simulink model "Astrolab_jumeaunumerique_2015a_v21"  (R2015b)
settings: Solver=ode3  SolverMode=SingleTasking  StartTime=0.0  StopTime=10  RelTol=1e-3
model workspace (MAT data in the model file):
  Freq = Simulink.Parameter
  Freq.DataType = 'auto'
  Freq.Units = 'auto'
  Freq.DocUnits = 'Hz'
libraries: powerlib_meascontrol x2
settings Model: Creator=utilisateur  LastModifiedBy=utilisateur
settings DataIOCC: LimitDataPoints=off  ReturnWorkspaceOutputs=on
settings DebuggingCC: SFUnexpectedBacktrackingDiag=error  SFNoUnconditionalDefaultTransitionDiag=error
settings HardwareCC: ProdWordSize=32  ProdHWDeviceType=Specified
settings ModelReferenceCC: PropagateSignalLabelsOutOfModel=on
settings SFSimCC: SimUseLocalCustomCode=on
settings RTWCC: RTWUseLocalCustomCode=on
settings GRTTargetCC: TargetLangStandard=C99 (ISO)
settings ConfigComp: CovMetricSettings=dwe  CovHtmlReporting=off  CovSaveCumulativeToWorkspaceVar=off  CovSaveSingleToWorkspaceVar=off  CovModelRefEnable=Off  CovExternalEMLEnable=on
settings ConfigurationSet: Description=Simscape Multibody

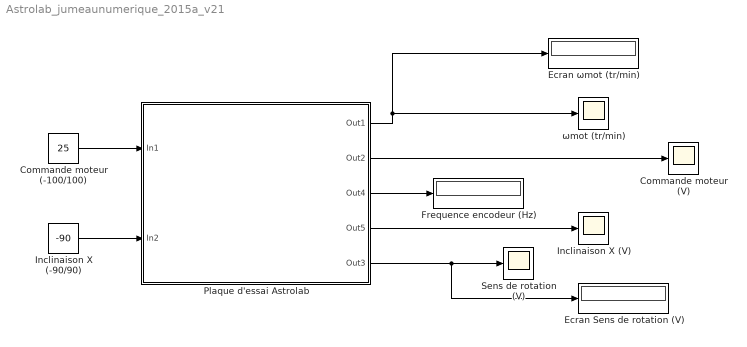
== system Astrolab_jumeaunumerique_2015a_v21 ==
  Commande moteur (-100/100) : Constant  Value=25
  Commande moteur (V) : Scope
  Ecran Sens de rotation (V) : Display
  Ecran ωmot (tr/min) : Display
  Frequence encodeur (Hz) : Display
  Inclinaison X (-90/90) : Constant  Value=-90
  Inclinaison X (V) : Scope
  Plaque d'essai Astrolab : Subsystem
      mask Display: image('plaque_astrolab.PNG')
  Sens de rotation (V) : Scope
  ωmot (tr/min) : Scope
  wires:
  Plaque d'essai Astrolab/1(Out1) -> Ecran ωmot (tr/min)/1, ωmot (tr/min)/1
  Plaque d'essai Astrolab/2(Out2) -> Commande moteur (V)/1
  Plaque d'essai Astrolab/3(Out4) -> Frequence encodeur (Hz)/1
  Plaque d'essai Astrolab/4(Out5) -> Inclinaison X (V)/1
  Inclinaison X (-90/90)/1 -> Plaque d'essai Astrolab/2(In2)
  Commande moteur (-100/100)/1 -> Plaque d'essai Astrolab/1(In1)
  Plaque d'essai Astrolab/5(Out3) -> Ecran Sens de rotation (V)/1, Sens de rotation (V)/1

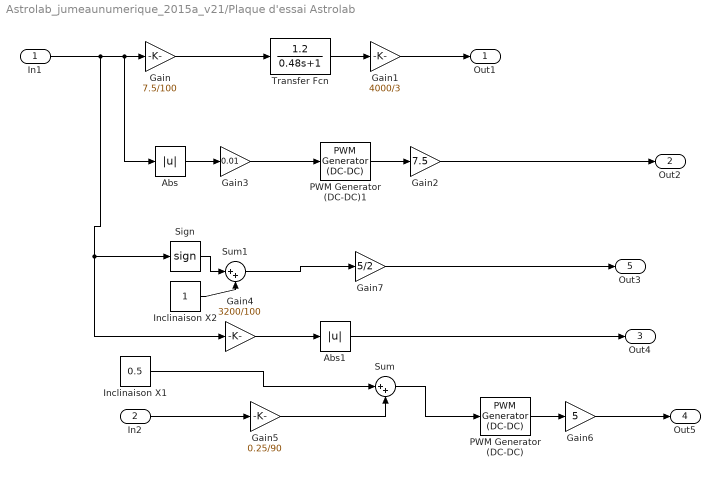
== system Astrolab_jumeaunumerique_2015a_v21/Plaque d'essai Astrolab ==
  In1 : Inport
  In2 : Inport  Port=2
  Abs : Abs
  Abs1 : Abs
  Gain : Gain  Gain=7.5/100
  Gain1 : Gain  Gain=4000/3
  Gain2 : Gain  Gain=7.5
  Gain3 : Gain  Gain=0.01
  Gain4 : Gain  Gain=3200/100
  Gain5 : Gain  Gain=0.25/90
  Gain6 : Gain  Gain=5
  Gain7 : Gain  Gain=5/2
  Inclinaison X1 : Constant  Value=0.5
  Inclinaison X2 : Constant
  PWM Generator (DC-DC) : powerlib_meascontrol/Pulse & Signal Generators/PWM Generator (DC-DC)  Fsw=1000  Ts=10e-5
  PWM Generator (DC-DC)1 : powerlib_meascontrol/Pulse & Signal Generators/PWM Generator (DC-DC)  Fsw=1000  Ts=10e-5
  Sign : Signum
  Sum : Sum  Inputs=|++
  Sum1 : Sum  Inputs=|++
  Transfer Fcn : TransferFcn  Numerator=[1.2]  Denominator=[0.48 1]
  Out1 : Outport
  Out2 : Outport  Port=2
  Out4 : Outport  Port=3
  Out5 : Outport  Port=4
  Out3 : Outport  Port=5
  wires:
  PWM Generator (DC-DC)1/1 -> Gain2/1
  In1/1 -> Sign/1, Gain4/1, Abs/1, Gain/1
  Gain2/1 -> Out2/1
  Gain3/1 -> PWM Generator (DC-DC)1/1
  Transfer Fcn/1 -> Gain1/1
  Sum/1 -> PWM Generator (DC-DC)/1
  PWM Generator (DC-DC)/1 -> Gain6/1
  Gain/1 -> Transfer Fcn/1
  In2/1 -> Gain5/1
  Inclinaison X1/1 -> Sum/1
  Gain5/1 -> Sum/2
  Gain1/1 -> Out1/1
  Gain4/1 -> Abs1/1
  Gain6/1 -> Out5/1
  Sum1/1 -> Gain7/1
  Sign/1 -> Sum1/1
  Gain7/1 -> Out3/1
  Inclinaison X2/1 -> Sum1/2
  Abs/1 -> Gain3/1
  Abs1/1 -> Out4/1
